simulink model "Lab6_1"  (R2014a)
settings: Solver=ode45  StartTime=0.0  StopTime=3.0  MaxStep=.001  RelTol=1e-3
settings Model: Creator=nandi2  LastModifiedBy=nandi2
settings DataIOCC: LimitDataPoints=off

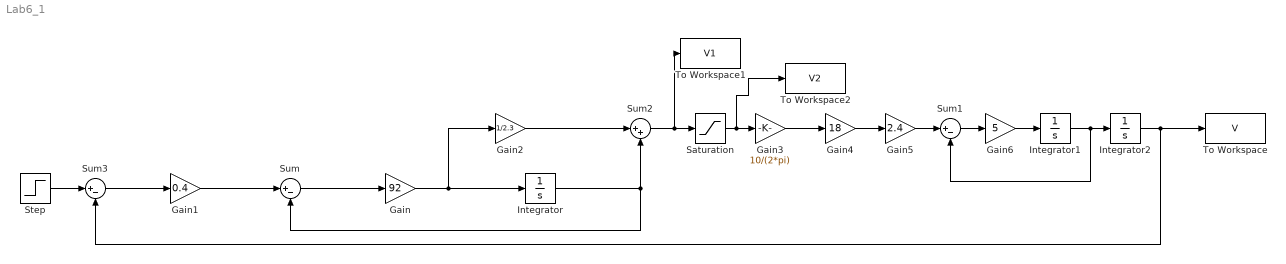
== system Lab6_1 ==
  Gain : Gain  Gain=92
  Gain1 : Gain  Gain=0.4
  Gain2 : Gain  Gain=1/2.3
  Gain3 : Gain  Gain=10/(2*pi)
  Gain4 : Gain  Gain=18
  Gain5 : Gain  Gain=2.4
  Gain6 : Gain  Gain=5
  Integrator : Integrator
  Integrator1 : Integrator
  Integrator2 : Integrator
  Saturation : Saturate  UpperLimit=10  LowerLimit=-10
  Step : Step  Time=0  After=50  SampleTime=0
  Sum : Sum  Inputs=|+-
  Sum1 : Sum  Inputs=|+-
  Sum2 : Sum  Inputs=|++
  Sum3 : Sum  Inputs=|+-
  To Workspace : ToWorkspace  VariableName=V  SampleTime=-1
  To Workspace1 : ToWorkspace  VariableName=V1  SampleTime=-1
  To Workspace2 : ToWorkspace  VariableName=V2  SampleTime=-1
  wires:
  Gain1/1 -> Sum/1
  Sum/1 -> Gain/1
  Gain2/1 -> Sum2/1
  Gain/1 -> Gain2/1, Integrator/1
  Sum3/1 -> Gain1/1
  Integrator/1 -> Sum2/2, Sum/2
  Gain3/1 -> Gain4/1
  Gain4/1 -> Gain5/1
  Gain5/1 -> Sum1/1
  Sum1/1 -> Gain6/1
  Gain6/1 -> Integrator1/1
  Integrator1/1 -> Sum1/2, Integrator2/1
  Integrator2/1 -> Sum3/2, To Workspace/1
  Step/1 -> Sum3/1
  Saturation/1 -> To Workspace2/1, Gain3/1
  Sum2/1 -> To Workspace1/1, Saturation/1
